simulink model "QRD_Ex3"  (R2025a)
settings: Solver=VariableStepAuto  StartTime=0.0  StopTime=10  RelTol=1e-3
InitFcn:
  | A = single(rand(8,8));
undefined symbols (not defined in the file): Column, major, S, static_input_Convolution_Stream_Ex1, Subsystem, vsva2197, xcvc1902
libraries: aieUtilities x2, aieSolver x1, vmcUtilities x1
settings Model: Creator=sdegala  LastModifiedBy=sdegala
settings ModelReferenceCC: EnableRefExpFcnMdlSchedulingChecks=on
settings RTWCC: GPUComputeCapability=3.5

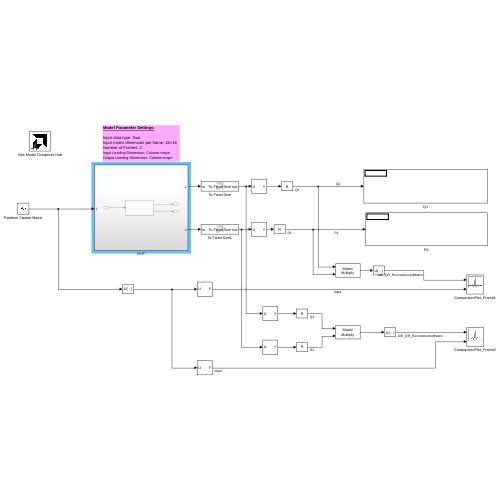
[thumbnail: Simulink's stored preview of the top-level diagram]
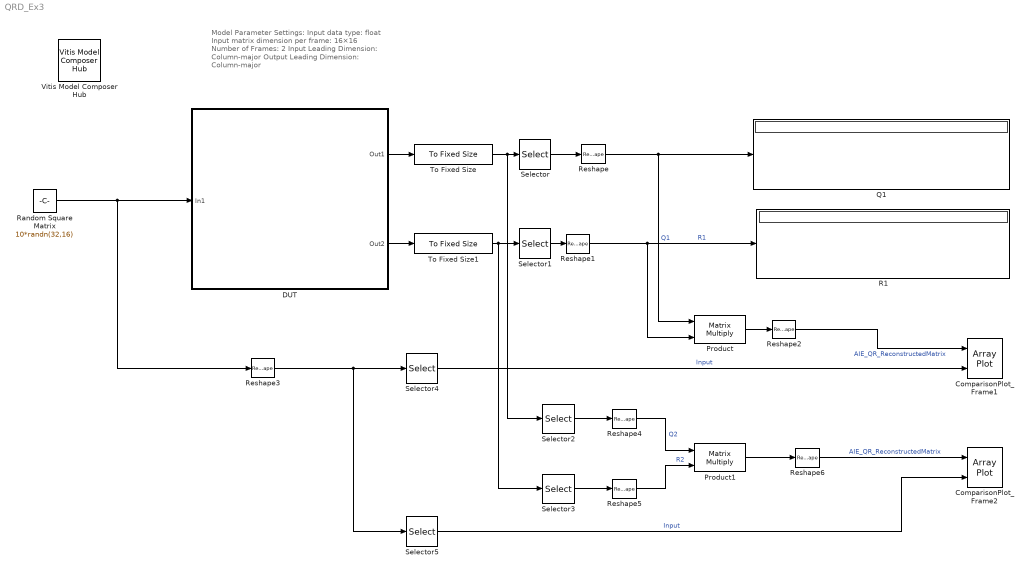
== system QRD_Ex3 ==
  note: Model Parameter Settings:
      |
      | Input data type: float
      | Input matrix dimension per frame: 16×16
      | Number of Frames: 2
      | Input Leading Dimension: Column-major
      | Output Leading Dimension: Column-major
  ComparisonPlot_Frame1 : ArrayPlot  NumInputPorts=2  WindowPosition=[6.000000,6.000000,1904.000000,1097.000000,]  ScopeFrameLocation=window  YLimits=[-30.6914 33.7477]  ShowLegend=on
  ComparisonPlot_Frame2 : ArrayPlot  NumInputPorts=2  WindowPosition=[6.000000,6.000000,1904.000000,1097.000000,]  ScopeFrameLocation=window  YLimits=[-29.8074 42.9771]  ShowLegend=on
  DUT : Subsystem
  Product : Product  Multiplication=Matrix(*)
  Product1 : Product  Multiplication=Matrix(*)
  Q1 : Display
  R1 : Display
  Random Square Matrix : Constant  Value=10*randn(32,16)  VectorParams1D=off  OutDataTypeStr=single  SampleTime=1
  Reshape{,1,4..5} (4 alike) : Reshape  OutputDimensionality=Customize  OutputDimensions=[16,16]
  Reshape2 : Reshape
  Reshape3 : Reshape
  Reshape6 : Reshape
  Selector : Selector  InputPortWidth=512  IndexOptions=Index vector (dialog)  Indices=1:1:256  OutputSizes=1
  Selector1 : Selector  InputPortWidth=512  IndexOptions=Index vector (dialog)  Indices=1:1:256  OutputSizes=1
  Selector2 : Selector  InputPortWidth=512  IndexOptions=Index vector (dialog)  Indices=257:1:512  OutputSizes=1
  Selector3 : Selector  InputPortWidth=512  IndexOptions=Index vector (dialog)  Indices=257:1:512  OutputSizes=1
  Selector4 : Selector  InputPortWidth=512  IndexOptions=Index vector (dialog)  Indices=1:1:256  OutputSizes=1
  Selector5 : Selector  InputPortWidth=512  IndexOptions=Index vector (dialog)  Indices=257:1:512  OutputSizes=1
  To Fixed Size : aieUtilities/To Fixed Size  Mode=Stop simulation when input variable-size signal is not full  OutputSize=Inherit: Same as input  CopyMethod=Buffer samples to form output  HasStatusOutput=on
  To Fixed Size1 : aieUtilities/To Fixed Size  Mode=Stop simulation when input variable-size signal is not full  OutputSize=Inherit: Same as input  CopyMethod=Buffer samples to form output  HasStatusOutput=on
  Vitis Model Composer Hub : vmcUtilities/Vitis Model Composer Hub  Tag=genX  CodeGeneration=off  SubsystemName=Subsystem  BlockHierPath=static_input_Convolution_Stream_Ex1/Subsystem  SubsystemType=AIENode  AIEArrayConfig=Use entire AIE array  StartColumn=1  NumberOfColumns=1  TargetDirectory=./code  exportDesign=on  analyzeDesign=off  validateDesignOnHw=off  ExportType=AI Engines  IpVendor=xilinx.com  IpLibrary=hls  IpVersion=1.0  IpHWLanguage=Verilog  AieCompilerOptions={}  AieSimulatorOptions={}  CreateTestbench=on  TestbenchStackSize=10  RunRtlSim=off  RunCSim=off  RunAieSim=off  enableSimulationTimeout=on  enableGraphIterations=on  AieSimTimeout=50000  AieGraphIterations=-1  RunAieSimProfiling=off  LaunchVitisAnalyzer=off  PlotOutput=off  RunX86Sim=off  X86SimTimeout=10  GenHwImage=off  GenLibadfXo=off  GenHwValidationCode=off  PlatformType=Not Specified  HwSystemType=Baremetal  HwValidationTarget=hw  ProjDevice=xcvc1902-vsva2197-1LP-e-S  ProjDevicePart=xcvc1902-vsva2197-1LP-e-S  AIEType=AIE  SamplePeriod=-1  ClockFrequency=200  DataPathParallelism=1  xilinxfamily=versalaicore  part=xcvc1902  speed=-1LP-e-S  package=vsva2197  directory=./netlist  testbench=off  incr_netlist=off  synthesis_tool=Vivado  clock_wrapper=Clock Enables  dbl_ovrd=According to Block Masks  dcm_input_clock_period=10  sysclk_period=10  simulink_period=1  eval_field=0  IPInfoJsonString="{\"DUTSubsystemName\":\"Subsystem\",\"AIESubsystem\":{\"SubsystemName\":\"Subsystem\",\"TargetDirectory\":\"./code\",\"AIEArrayConfig\":\"Use entire AIE array\",\"StartColumn\":\"0\",\"NumberOfColumns\":\"1\"},\"SubsystemTag\":\"AIENode\"}"  LogFileName=/tmp/CR-1250814/code/model_composer.log  NThreads=4  IPConfigFile=/tmp/vmctmp-13380004059271250980/static_input_Convolution_Stream_Ex1_ipconfig.json
  wires:
  To Fixed Size/1 -> Selector2/1, Selector/1
  Reshape/1 -> Q1/1, Product/1  "Q1"
  To Fixed Size1/1 -> Selector3/1, Selector1/1
  Reshape1/1 -> R1/1, Product/2  "R1"
  Product/1 -> Reshape2/1
  Reshape2/1 -> ComparisonPlot_Frame1/1  "AIE_QR_ReconstructedMatrix"
  Reshape3/1 -> Selector5/1, Selector4/1
  DUT/1(Out1) -> To Fixed Size/1
  DUT/2(Out2) -> To Fixed Size1/1
  Random Square Matrix/1 -> DUT/1(In1), Reshape3/1
  Selector/1 -> Reshape/1
  Selector1/1 -> Reshape1/1
  Selector2/1 -> Reshape4/1
  Selector3/1 -> Reshape5/1
  Reshape4/1 -> Product1/1  "Q2"
  Reshape5/1 -> Product1/2  "R2"
  Product1/1 -> Reshape6/1
  Reshape6/1 -> ComparisonPlot_Frame2/1  "AIE_QR_ReconstructedMatrix"
  Selector4/1 -> ComparisonPlot_Frame1/2  "Input"
  Selector5/1 -> ComparisonPlot_Frame2/2  "Input"

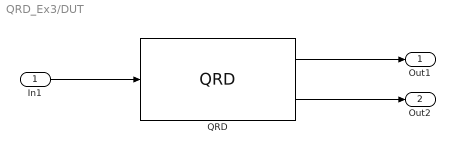
== system QRD_Ex3/DUT ==
  In1 : Inport
  QRD : aieSolver/QRD  AIE_VARIANT=1  data_type=float  row_dimension=16  cols_dimension=16  num_frames=2  casc_length=1  dim_a_leading=Column-major(0)  dim_q_leading=Column-major(0)  dim_r_leading=Column-major(0)  blockJsonConstraints=[]  blockJsonConstraintsInternal=[]  spec=vmc_qrd.json  SerializedMaskParamNames=[]  SerializedMaskParamValues=[]  SerializedMaskParamVisibilities=[]  block_type=QRD  SerializedMaskParamDataypes=uint|typename|uint|uint|uint|uint|uint|uint|uint  SerializedMaskParamEnumStrArr=0|0|0|0|0|0|Column-major(0),Row-major(1)|Column-major(0),Row-major(1)|Column-major(0),Row-major(1)  SerializedMaskParamEnumValArr=0|0|0|0|0|0|0,1|0,1|0,1  SerializedMaskParamVectorArr=0|0|0|0|0|0|0|0|0  SerializedMaskParamKeys=AIE_VARIANT|TT_DATA|TP_DIM_ROWS|TP_DIM_COLS|TP_NUM_FRAMES|TP_CASC_LEN|TP_DIM_A_LEADING|TP_DIM_Q_LEADING|TP_DIM_R_LEADING
  Out1 : Outport
  Out2 : Outport  Port=2
  wires:
  In1/1 -> QRD/1
  QRD/2 -> Out2/1
  QRD/1 -> Out1/1
